simulink model "Task_8_NL_Rleak"  (R2015a)
settings: Solver=ode45  StartTime=0.0  StopTime=10.0  RelTol=1e-3
libraries: simulink x2
settings Model: Creator=Farhan Fuad  LastModifiedBy=Farhan Fuad

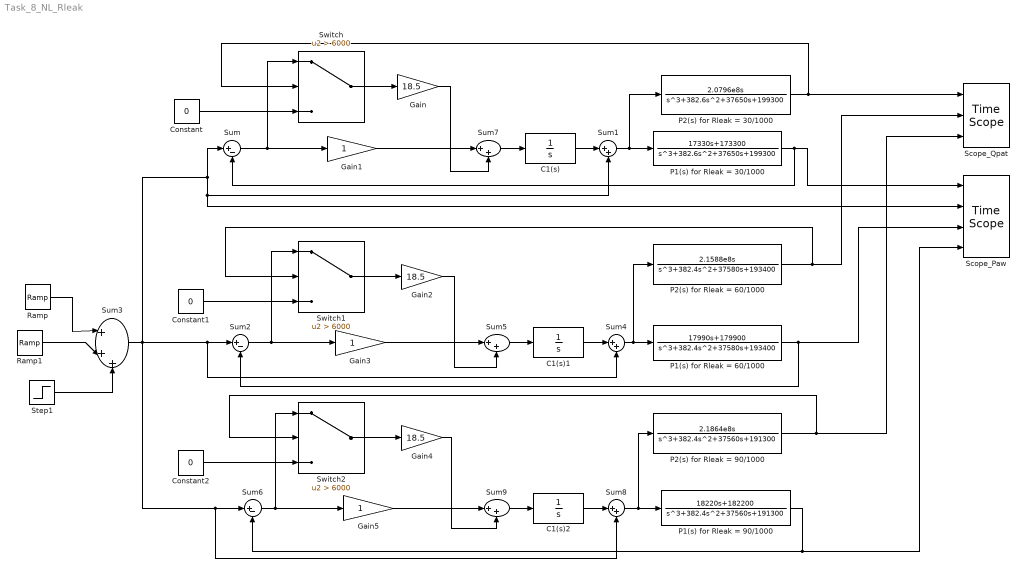
== system Task_8_NL_Rleak ==
  C1(s) : TransferFcn  Numerator=[0 1]  Denominator=[1 0]
  C1(s)1 : TransferFcn  Numerator=[0 1]  Denominator=[1 0]
  C1(s)2 : TransferFcn  Numerator=[0 1]  Denominator=[1 0]
  Constant : Constant  Value=0
  Constant1 : Constant  Value=0
  Constant2 : Constant  Value=0
  Gain : Gain  Gain=18.5
  Gain1 : Gain
  Gain2 : Gain  Gain=18.5
  Gain3 : Gain
  Gain4 : Gain  Gain=18.5
  Gain5 : Gain
  P1(s) for Rleak = 30/1000 : TransferFcn  Numerator=[0 0 17330 173300]  Denominator=[1 382.6 37650 199300]
  P1(s) for Rleak = 60/1000 : TransferFcn  Numerator=[0 0 17990 179900]  Denominator=[1 382.4 37580 193400]
  P1(s) for Rleak = 90/1000 : TransferFcn  Numerator=[0 0 18220 182200]  Denominator=[1 382.4 37560 191300]
  P2(s) for Rleak = 30/1000 : TransferFcn  Numerator=[0 0 2.0796e8 0]  Denominator=[1 382.6 37650 199300]
  P2(s) for Rleak = 60/1000 : TransferFcn  Numerator=[0 0 2.1588e8 0]  Denominator=[1 382.4 37580 193400]
  P2(s) for Rleak = 90/1000 : TransferFcn  Numerator=[0 0 2.1864e8 0]  Denominator=[1 382.4 37560 191300]
  Ramp : simulink/Sources/Ramp  slope=64.865  start=1  X0=0
  Ramp1 : simulink/Sources/Ramp  slope=-64.865  start=1.23125  X0=0
  Scope_Paw : TimeScope  NumInputPorts=4
  Scope_Qpat : TimeScope  NumInputPorts=3
  Step1 : Step  Time=5  After=-15  SampleTime=0
  Sum : Sum  Inputs=|+-
  Sum{1,4..5,7..9} (6 alike) : Sum  Inputs=|++
  Sum2 : Sum  Inputs=|+-
  Sum3 : Sum  Inputs=|+++
  Sum6 : Sum  Inputs=|+-
  Switch : Switch  Criteria=u2 > Threshold  Threshold=6000
  Switch1 : Switch  Criteria=u2 > Threshold  Threshold=6000
  Switch2 : Switch  Criteria=u2 > Threshold  Threshold=6000
  wires:
  Ramp/1 -> Sum3/1
  Ramp1/1 -> Sum3/2
  P1(s) for Rleak = 30/1000/1 -> Scope_Paw/1, Sum/2
  Sum1/1 -> P1(s) for Rleak = 30/1000/1, P2(s) for Rleak = 30/1000/1
  Step1/1 -> Sum3/3
  C1(s)/1 -> Sum1/1
  Switch/1 -> Gain/1
  Sum/1 -> Gain1/1, Switch/1
  P2(s) for Rleak = 30/1000/1 -> Switch/2, Scope_Qpat/1
  Gain1/1 -> Sum7/1
  Sum7/1 -> C1(s)/1
  Gain/1 -> Sum7/2
  Constant/1 -> Switch/3
  Sum4/1 -> P1(s) for Rleak = 60/1000/1, P2(s) for Rleak = 60/1000/1
  C1(s)1/1 -> Sum4/1
  Switch1/1 -> Gain2/1
  Sum2/1 -> Gain3/1, Switch1/1
  Gain3/1 -> Sum5/1
  Sum5/1 -> C1(s)1/1
  Gain2/1 -> Sum5/2
  Constant1/1 -> Switch1/3
  P2(s) for Rleak = 60/1000/1 -> Scope_Qpat/2, Switch1/2
  P1(s) for Rleak = 60/1000/1 -> Sum2/2, Scope_Paw/3
  P1(s) for Rleak = 90/1000/1 -> Scope_Paw/4, Sum6/2
  Sum8/1 -> P1(s) for Rleak = 90/1000/1, P2(s) for Rleak = 90/1000/1
  C1(s)2/1 -> Sum8/1
  Switch2/1 -> Gain4/1
  Sum6/1 -> Gain5/1, Switch2/1
  P2(s) for Rleak = 90/1000/1 -> Scope_Qpat/3, Switch2/2
  Sum3/1 -> Sum8/2, Sum6/1, Scope_Paw/2, Sum1/2, Sum/1, Sum4/2, Sum2/1
  Gain5/1 -> Sum9/1
  Sum9/1 -> C1(s)2/1
  Gain4/1 -> Sum9/2
  Constant2/1 -> Switch2/3
